simulink model "ControlledVehicleSystem_PID"  (R2019b)
settings: Solver=FixedStepAuto  StartTime=0.0  StopTime=15  FixedStep=0.005  RelTol=1e-3
model workspace (MAT data in the model file):
  I_a = 2.25
  I_f = 2.25
  Kda = 1
  Kdf = 1
  Kpa = 1
  Kpf = 1
  Kpv = 25
  Rfl = 0.1
  Rfr = 0.1
  Rrl = 0.1
  Rrr = 0.1
  Tla = 0.6
  Tlf = 0.6
  coeffDerivative = 1
  m_v = 200
undefined symbols (not defined in the file): DiscIntNeverNeededParam, sigbuilder_block
libraries: simulink x8
settings Model: Creator=arfbj  LastModifiedBy=frqbv

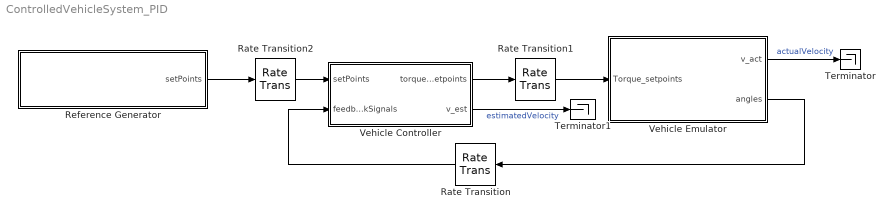
== system ControlledVehicleSystem_PID ==
  Rate Transition : RateTransition
  Rate Transition1 : RateTransition
  Rate Transition2 : RateTransition
  Reference Generator : Subsystem
  Terminator : Terminator
  Terminator1 : Terminator
  Vehicle Controller : Subsystem
  Vehicle Emulator : Subsystem
  wires:
  Vehicle Emulator/2(angles) -> Rate Transition/1
  Reference Generator/1(setPoints) -> Rate Transition2/1
  Vehicle Controller/1(torqueSetpoints) -> Rate Transition1/1
  Vehicle Emulator/1(v_act) -> Terminator/1  "actualVelocity"
  Vehicle Controller/2(v_est) -> Terminator1/1  "estimatedVelocity"
  Rate Transition/1 -> Vehicle Controller/2(feedbackSignals)
  Rate Transition1/1 -> Vehicle Emulator/1(Torque_setpoints)
  Rate Transition2/1 -> Vehicle Controller/1(setPoints)

== system ControlledVehicleSystem_PID/Reference Generator ==
  Bus Creator : BusCreator  Inputs=3
  Signal Builder : Subsystem  Tag=STV Subsys  LoadFcn=sigbuilder_block('load');  StartFcn=sigbuilder_block('start');  StopFcn=sigbuilder_block('stop');  ClipboardFcn=sigbuilder_block('clipboard');  mask(Sigbuilder block){tuvar=[0:10]}
      mask help: Simulink:masks:SigbuilderBlock_MD
      mask init:
      | if ~strcmp(get_param(bdroot(gcbh),'SimulationStatus'),'stopped') tuvar = sigbuilder_block('maskInit'); end
      settings: CopyFcn=sigbuilder_block('copy');  DeleteFcn=sigbuilder_block('delete');  ModelCloseFcn=sigbuilder_block('modelClose');  PreSaveFcn=sigbuilder_block('preSave');  PauseFcn=sigbuilder_block('pause');  ContinueFcn=sigbuilder_block('continue');  NameChangeFcn=sigbuilder_block('namechange');  OpenFcn=sigbuilder_block('open',[1521.6 55.8 550.2 362.4 ]);  CloseFcn=sigbuilder_block('close');
      mask Display: plot(0, 0, 100, 100,[2, 2, 32, 32, 2], [68, 8, 8, 68, 68],[32, 2], [38, 38], [32, 19, 2],[53, 60, 44], [32, 17, 17, 2],[16, 16, 31, 31]);txt = getActiveGroup(gcbh);text(2, 100, txt,'verticalAlignment', 'top');
  setPoints : Outport
  wires:
  Signal Builder/1(v_set) -> Bus Creator/1  "v_set"
  Signal Builder/2(delta_f_set) -> Bus Creator/2  "delta_f_set"
  Signal Builder/3(delta_a_set) -> Bus Creator/3  "delta_a_set"
  Bus Creator/1 -> setPoints/1

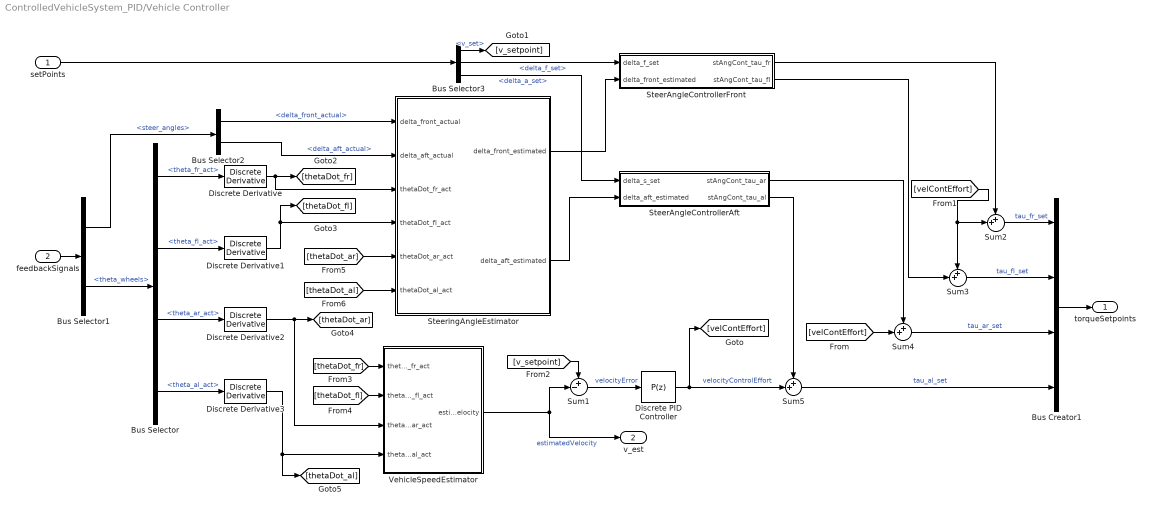
== system ControlledVehicleSystem_PID/Vehicle Controller ==
  setPoints : Inport
  feedbackSignals : Inport  Port=2
  Bus Creator1 : BusCreator  Inputs=4
  Bus Selector : BusSelector  OutputSignals=theta_fr_act,theta_fl_act,theta_ar_act,theta_al_act
  Bus Selector1 : BusSelector  OutputSignals=steer_angles,theta_wheels
  Bus Selector2 : BusSelector  OutputSignals=delta_front_actual,delta_aft_actual
  Bus Selector3 : BusSelector  OutputSignals=v_set,delta_f_set,delta_a_set
  Discrete Derivative{,1..3} (4 alike) : simulink/Discrete/Discrete Derivative  gainval=1.0  ICPrevScaledInput=0.0  OutMin=[]  OutMax=[]  OutDataType=fixdt(1, 16)  OutScaling=2^-10  DoSatur=off
  Discrete PID Controller : simulink/Continuous/PID Controller  Controller=P  Form=Parallel  TimeDomain=Discrete-time  SampleTime=-1  IntegratorMethod=Forward Euler  FilterMethod=Forward Euler  ControllerParametersSource=internal  P=20  I=1  D=5  UseFilter=on  N=100  TunerSelectOption=Transfer Function Based (PID Tuner App)  InitialConditionSource=internal  InitialConditionForIntegrator=0  InitialConditionForFilter=0  DifferentiatorICPrevScaledInput=0  ExternalReset=none  TrackingMode=off  Kt=1  LimitOutput=off  UpperSaturationLimit=inf  LowerSaturationLimit=-inf  LinearizeAsGain=off  AntiWindupMode=none  Kb=1  POutMin=[]  POutMax=[]  IOutMin=[]  IOutMax=[]  DOutMin=[]  DOutMax=[]  NOutMin=[]  NOutMax=[]  SumOutMin=[]  SumOutMax=[]  SaturationOutMin=[]  SaturationOutMax=[]  PParamMin=[]  PParamMax=[]  IParamMin=[]  IParamMax=[]  DParamMin=[]  DParamMax=[]  NParamMin=[]  NParamMax=[]  KbParamMin=[]  KbParamMax=[]  KtParamMin=[]  KtParamMax=[]  KbOutMin=[]  KbOutMax=[]  KtOutMin=[]  KtOutMax=[]  IntegratorOutMin=[]  IntegratorOutMax=[]  FilterOutMin=[]  FilterOutMax=[]  SumI1OutMin=[]  SumI1OutMax=[]  SumI2OutMin=[]  SumI2OutMax=[]  SumI3OutMin=[]  SumI3OutMax=[]  SumI4OutMin=[]  SumI4OutMax=[]  SumDOutMin=[]  SumDOutMax=[]  DifferentiatorOutMin=[]  DifferentiatorOutMax=[]  FilterDiffOutCoefMin=[]  FilterDiffOutCoefMax=[]  ReciprocalOutMin=[]  ReciprocalOutMax=[]  SumDenOutMin=[]  SumDenOutMax=[]  SumNumOutMin=[]  SumNumOutMax=[]  DivideOutMin=[]  DivideOutMax=[]  IntegratorContinuousStateAttributes=''  IntegratorStateMustResolveToSignalObject=off  IntegratorRTWStateStorageClass=Auto  FilterContinuousStateAttributes=''  FilterStateMustResolveToSignalObject=off  FilterRTWStateStorageClass=Auto  ParallelPVariant=InternalParameters  IdealPVariant=Disabled  IVariant=Disabled  DVariant=Disabled  IntegratorVariant=Disabled  SatVariant=Disabled  AWVariant=Disabled  PCopyVariant=Disabled  TRVariant=Disabled  FdbkBlocksVariant=Forward  IdealPFdbkVariant=Disabled  SatFdbkVariant=Disabled  DerivativeFilterVariant=Disabled  NVariant=Disabled  NCopyVariant=Disabled_SignalSpec  FilterICVariant=Disabled  IntegratorICVariant=Disabled  ExternalResetVariant=Disabled  TRSumVariant=Passthrough  SumFdbkVariant=Disabled  SumVariant=Passthrough_P
  SteerAngleControllerAft : Subsystem
  SteerAngleControllerFront : Subsystem
  SteeringAngleEstimator : Subsystem
  Sum1 : Sum  Inputs=+-|
  Sum{2..5} (4 alike) : Sum  Inputs=++|
  VehicleSpeedEstimator : Subsystem
  torqueSetpoints : Outport
  v_est : Outport  Port=2
  wires:
  feedbackSignals/1 -> Bus Selector1/1
  Bus Selector1/2 -> Bus Selector/1  "<theta_wheels>"
  Bus Selector1/1 -> Bus Selector2/1  "<steer_angles>"
  Bus Selector/1 -> Discrete Derivative/1  "<theta_fr_act>"
  Bus Selector/2 -> Discrete Derivative1/1  "<theta_fl_act>"
  Bus Selector/3 -> Discrete Derivative2/1  "<theta_ar_act>"
  Bus Selector/4 -> Discrete Derivative3/1  "<theta_al_act>"
  Discrete Derivative/1 -> [thetaDot_fr], SteeringAngleEstimator/3(thetaDot_fr_act)
  Discrete Derivative2/1 -> VehicleSpeedEstimator/3(thetaDot_ar_act), [thetaDot_ar]
  Discrete Derivative3/1 -> [thetaDot_al], VehicleSpeedEstimator/4(thetaDot_al_act)
  Discrete Derivative1/1 -> [thetaDot_fl], SteeringAngleEstimator/4(thetaDot_fl_act)
  Bus Selector2/1 -> SteeringAngleEstimator/1(delta_front_actual)  "<delta_front_actual>"
  Bus Selector2/2 -> SteeringAngleEstimator/2(delta_aft_actual)  "<delta_aft_actual>"
  SteeringAngleEstimator/1(delta_front_estimated) -> SteerAngleControllerFront/2(delta_front_estimated)
  Bus Creator1/1 -> torqueSetpoints/1
  VehicleSpeedEstimator/1(estimatedVelocity) -> v_est/1, Sum1/2  "estimatedVelocity"
  Sum1/1 -> Discrete PID Controller/1  "velocityError"
  Sum4/1 -> Bus Creator1/3  "tau_ar_set"
  Sum5/1 -> Bus Creator1/4  "tau_al_set"
  Sum3/1 -> Bus Creator1/2  "tau_fl_set"
  Sum2/1 -> Bus Creator1/1  "tau_fr_set"
  setPoints/1 -> Bus Selector3/1
  [v_setpoint] -> Sum1/1
  Bus Selector3/2 -> SteerAngleControllerFront/1(delta_f_set)  "<delta_f_set>"
  SteeringAngleEstimator/2(delta_aft_estimated) -> SteerAngleControllerAft/2(delta_aft_estimated)
  Bus Selector3/3 -> SteerAngleControllerAft/1(delta_s_set)  "<delta_a_set>"
  SteerAngleControllerFront/1(stAngCont_tau_fr) -> Sum2/1
  SteerAngleControllerFront/2(stAngCont_tau_fl) -> Sum3/2
  SteerAngleControllerAft/1(stAngCont_tau_ar) -> Sum4/1
  SteerAngleControllerAft/2(stAngCont_tau_al) -> Sum5/1
  Discrete PID Controller/1 -> [velContEffort], Sum5/2  "velocityControlEffort"
  [velContEffort] -> Sum4/2
  [velContEffort] -> Sum3/1, Sum2/2
  Bus Selector3/1 -> [v_setpoint]  "<v_set>"
  [thetaDot_fr] -> VehicleSpeedEstimator/1(thetaDot_fr_act)
  [thetaDot_fl] -> VehicleSpeedEstimator/2(thetaDot_fl_act)
  [thetaDot_ar] -> SteeringAngleEstimator/5(thetaDot_ar_act)
  [thetaDot_al] -> SteeringAngleEstimator/6(thetaDot_al_act)

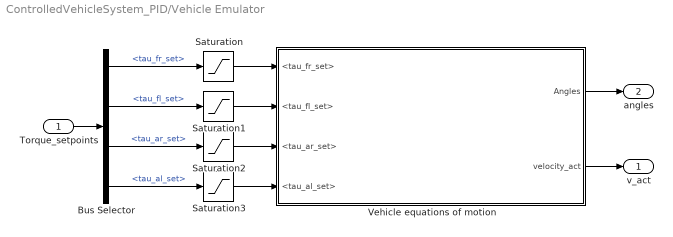
== system ControlledVehicleSystem_PID/Vehicle Emulator ==
  Torque_setpoints : Inport
  Bus Selector : BusSelector  OutputSignals=tau_fr_set,tau_fl_set,tau_ar_set,tau_al_set
  Saturation{,1..3} (4 alike) : Saturate  UpperLimit=5  LowerLimit=-5
  Vehicle equations of motion : Subsystem
  v_act : Outport
  angles : Outport  Port=2
  wires:
  Torque_setpoints/1 -> Bus Selector/1
  Bus Selector/2 -> Saturation1/1  "<tau_fl_set>"
  Bus Selector/1 -> Saturation/1  "<tau_fr_set>"
  Bus Selector/3 -> Saturation2/1  "<tau_ar_set>"
  Bus Selector/4 -> Saturation3/1  "<tau_al_set>"
  Vehicle equations of motion/1(Angles) -> angles/1
  Vehicle equations of motion/2(velocity_act) -> v_act/1
  Saturation/1 -> Vehicle equations of motion/1(<tau_fr_set>)
  Saturation1/1 -> Vehicle equations of motion/2(<tau_fl_set>)
  Saturation2/1 -> Vehicle equations of motion/3(<tau_ar_set>)
  Saturation3/1 -> Vehicle equations of motion/4(<tau_al_set>)

== system ControlledVehicleSystem_PID/Reference Generator/Signal Builder ==
  Demux : Demux  Tag=STV Demux  Outputs=3
  FromWs : FromWorkspace  Tag=STV FromWs  VariableName=tuvar  SampleTime=0
      SigBuilderData=|
      | common.afterFinalStr = 'Extrapolate'
      | common.sampleTime = 0
      | dataSet.timeRange = [0 10]
      | dataSet.name = 'Group 1'
      | sbobj.Groups.Name = 'Group 1'
      | sbobj.Groups.Signals(1).Name = 'v_set'
      | sbobj.Groups.Signals(1).XData = [0 1 3 5 6 8 9 10]
      | sbobj.Groups.Signals(1).YData = [-0.005 -0.00375 1 1 0.5 0.5 0 0]
      | sbobj.Groups.Signals(2).Name = 'delta_f_set'
      | sbobj.Groups.Signals(2).XData = [0 10]
      | sbobj.Groups.Signals(2).YData = [0 0]
      | sbobj.Groups.Signals(3).Name = 'delta_a_set'
      | sbobj.Groups.Signals(3).XData = [0 10]
      | sbobj.Groups.Signals(3).YData = [0 0]
  v_set : Outport  Tag=STV Outport
  delta_f_set : Outport  Tag=STV Outport  Port=2
  delta_a_set : Outport  Tag=STV Outport  Port=3
  wires:
  Demux/1 -> v_set/1
  FromWs/1 -> Demux/1
  Demux/2 -> delta_f_set/1
  Demux/3 -> delta_a_set/1

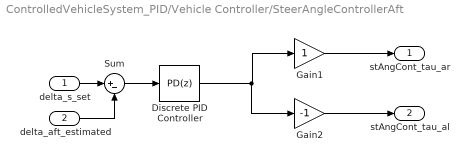
== system ControlledVehicleSystem_PID/Vehicle Controller/SteerAngleControllerAft ==
  delta_s_set : Inport
  delta_aft_estimated : Inport  Port=2
  Discrete PID Controller : simulink/Continuous/PID Controller  Controller=PD  Form=Parallel  TimeDomain=Discrete-time  SampleTime=-1  IntegratorMethod=Forward Euler  FilterMethod=Forward Euler  ControllerParametersSource=internal  P=1  I=1  D=1  UseFilter=on  N=100  TunerSelectOption=Transfer Function Based (PID Tuner App)  InitialConditionSource=internal  InitialConditionForIntegrator=0  InitialConditionForFilter=0  DifferentiatorICPrevScaledInput=0  ExternalReset=none  TrackingMode=off  Kt=1  LimitOutput=off  UpperSaturationLimit=inf  LowerSaturationLimit=-inf  LinearizeAsGain=off  AntiWindupMode=none  Kb=1  POutMin=[]  POutMax=[]  IOutMin=[]  IOutMax=[]  DOutMin=[]  DOutMax=[]  NOutMin=[]  NOutMax=[]  SumOutMin=[]  SumOutMax=[]  SaturationOutMin=[]  SaturationOutMax=[]  PParamMin=[]  PParamMax=[]  IParamMin=[]  IParamMax=[]  DParamMin=[]  DParamMax=[]  NParamMin=[]  NParamMax=[]  KbParamMin=[]  KbParamMax=[]  KtParamMin=[]  KtParamMax=[]  KbOutMin=[]  KbOutMax=[]  KtOutMin=[]  KtOutMax=[]  IntegratorOutMin=[]  IntegratorOutMax=[]  FilterOutMin=[]  FilterOutMax=[]  SumI1OutMin=[]  SumI1OutMax=[]  SumI2OutMin=[]  SumI2OutMax=[]  SumI3OutMin=[]  SumI3OutMax=[]  SumI4OutMin=[]  SumI4OutMax=[]  SumDOutMin=[]  SumDOutMax=[]  DifferentiatorOutMin=[]  DifferentiatorOutMax=[]  FilterDiffOutCoefMin=[]  FilterDiffOutCoefMax=[]  ReciprocalOutMin=[]  ReciprocalOutMax=[]  SumDenOutMin=[]  SumDenOutMax=[]  SumNumOutMin=[]  SumNumOutMax=[]  DivideOutMin=[]  DivideOutMax=[]  IntegratorContinuousStateAttributes=''  IntegratorStateMustResolveToSignalObject=off  IntegratorRTWStateStorageClass=Auto  FilterContinuousStateAttributes=''  FilterStateMustResolveToSignalObject=off  FilterRTWStateStorageClass=Auto  ParallelPVariant=InternalParameters  IdealPVariant=Disabled  IVariant=Disabled  DVariant=InternalParameters  IntegratorVariant=Disabled  SatVariant=Disabled  AWVariant=Disabled  PCopyVariant=Disabled  TRVariant=Disabled  FdbkBlocksVariant=Forward  IdealPFdbkVariant=Disabled  SatFdbkVariant=Disabled  DerivativeFilterVariant=ForwardEulerFilter  NVariant=InternalParameters  NCopyVariant=Disabled  FilterICVariant=InternalICsFilter  IntegratorICVariant=Disabled  ExternalResetVariant=Disabled  TRSumVariant=Passthrough  SumFdbkVariant=Disabled  SumVariant=Sum_PD
  Gain1 : Gain
  Gain2 : Gain  Gain=-1
  Sum : Sum  Inputs=|+-
  stAngCont_tau_ar : Outport
  stAngCont_tau_al : Outport  Port=2
  wires:
  Gain1/1 -> stAngCont_tau_ar/1
  Gain2/1 -> stAngCont_tau_al/1
  delta_s_set/1 -> Sum/1
  Sum/1 -> Discrete PID Controller/1
  delta_aft_estimated/1 -> Sum/2
  Discrete PID Controller/1 -> Gain2/1, Gain1/1

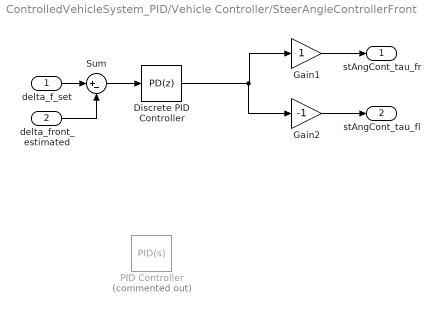
== system ControlledVehicleSystem_PID/Vehicle Controller/SteerAngleControllerFront ==
  delta_f_set : Inport
  delta_front_estimated : Inport  Port=2
  Discrete PID Controller : simulink/Continuous/PID Controller  Controller=PD  Form=Parallel  TimeDomain=Discrete-time  SampleTime=-1  IntegratorMethod=Forward Euler  FilterMethod=Forward Euler  ControllerParametersSource=internal  P=1  I=0  D=1  UseFilter=on  N=100  TunerSelectOption=Transfer Function Based (PID Tuner App)  InitialConditionSource=internal  InitialConditionForIntegrator=0  InitialConditionForFilter=0  DifferentiatorICPrevScaledInput=0  ExternalReset=none  TrackingMode=off  Kt=1  LimitOutput=off  UpperSaturationLimit=inf  LowerSaturationLimit=-inf  LinearizeAsGain=off  AntiWindupMode=none  Kb=1  POutMin=[]  POutMax=[]  IOutMin=[]  IOutMax=[]  DOutMin=[]  DOutMax=[]  NOutMin=[]  NOutMax=[]  SumOutMin=[]  SumOutMax=[]  SaturationOutMin=[]  SaturationOutMax=[]  PParamMin=[]  PParamMax=[]  IParamMin=[]  IParamMax=[]  DParamMin=[]  DParamMax=[]  NParamMin=[]  NParamMax=[]  KbParamMin=[]  KbParamMax=[]  KtParamMin=[]  KtParamMax=[]  KbOutMin=[]  KbOutMax=[]  KtOutMin=[]  KtOutMax=[]  IntegratorOutMin=[]  IntegratorOutMax=[]  FilterOutMin=[]  FilterOutMax=[]  SumI1OutMin=[]  SumI1OutMax=[]  SumI2OutMin=[]  SumI2OutMax=[]  SumI3OutMin=[]  SumI3OutMax=[]  SumI4OutMin=[]  SumI4OutMax=[]  SumDOutMin=[]  SumDOutMax=[]  DifferentiatorOutMin=[]  DifferentiatorOutMax=[]  FilterDiffOutCoefMin=[]  FilterDiffOutCoefMax=[]  ReciprocalOutMin=[]  ReciprocalOutMax=[]  SumDenOutMin=[]  SumDenOutMax=[]  SumNumOutMin=[]  SumNumOutMax=[]  DivideOutMin=[]  DivideOutMax=[]  IntegratorContinuousStateAttributes=''  IntegratorStateMustResolveToSignalObject=off  IntegratorRTWStateStorageClass=Auto  FilterContinuousStateAttributes=''  FilterStateMustResolveToSignalObject=off  FilterRTWStateStorageClass=Auto  ParallelPVariant=InternalParameters  IdealPVariant=Disabled  IVariant=Disabled  DVariant=InternalParameters  IntegratorVariant=Disabled  SatVariant=Disabled  AWVariant=Disabled  PCopyVariant=Disabled  TRVariant=Disabled  FdbkBlocksVariant=Forward  IdealPFdbkVariant=Disabled  SatFdbkVariant=Disabled  DerivativeFilterVariant=ForwardEulerFilter  NVariant=InternalParameters  NCopyVariant=Disabled  FilterICVariant=InternalICsFilter  IntegratorICVariant=Disabled  ExternalResetVariant=Disabled  TRSumVariant=Passthrough  SumFdbkVariant=Disabled  SumVariant=Sum_PD
  Gain1 : Gain
  Gain2 : Gain  Gain=-1
  PID Controller : simulink/Continuous/PID Controller  Commented=on  Controller=PID  Form=Parallel  TimeDomain=Continuous-time  SampleTime=-1  IntegratorMethod=Forward Euler  FilterMethod=Forward Euler  ControllerParametersSource=internal  P=Kpf  I=1  D=Kdf  UseFilter=on  N=100  TunerSelectOption=Transfer Function Based (PID Tuner App)  InitialConditionSource=internal  InitialConditionForIntegrator=0  InitialConditionForFilter=0  DifferentiatorICPrevScaledInput=0  ExternalReset=none  TrackingMode=off  Kt=1  LimitOutput=off  UpperSaturationLimit=inf  LowerSaturationLimit=-inf  LinearizeAsGain=on  AntiWindupMode=none  Kb=1  POutMin=[]  POutMax=[]  IOutMin=[]  IOutMax=[]  DOutMin=[]  DOutMax=[]  NOutMin=[]  NOutMax=[]  SumOutMin=[]  SumOutMax=[]  SaturationOutMin=[]  SaturationOutMax=[]  PParamMin=[]  PParamMax=[]  IParamMin=[]  IParamMax=[]  DParamMin=[]  DParamMax=[]  NParamMin=[]  NParamMax=[]  KbParamMin=[]  KbParamMax=[]  KtParamMin=[]  KtParamMax=[]  KbOutMin=[]  KbOutMax=[]  KtOutMin=[]  KtOutMax=[]  IntegratorOutMin=[]  IntegratorOutMax=[]  FilterOutMin=[]  FilterOutMax=[]  SumI1OutMin=[]  SumI1OutMax=[]  SumI2OutMin=[]  SumI2OutMax=[]  SumI3OutMin=[]  SumI3OutMax=[]  SumI4OutMin=[]  SumI4OutMax=[]  SumDOutMin=[]  SumDOutMax=[]  DifferentiatorOutMin=[]  DifferentiatorOutMax=[]  FilterDiffOutCoefMin=[]  FilterDiffOutCoefMax=[]  ReciprocalOutMin=[]  ReciprocalOutMax=[]  SumDenOutMin=[]  SumDenOutMax=[]  SumNumOutMin=[]  SumNumOutMax=[]  DivideOutMin=[]  DivideOutMax=[]  IntegratorContinuousStateAttributes=''  IntegratorStateMustResolveToSignalObject=off  IntegratorRTWStateStorageClass=Auto  FilterContinuousStateAttributes=''  FilterStateMustResolveToSignalObject=off  FilterRTWStateStorageClass=Auto  ParallelPVariant=InternalParameters  IdealPVariant=Disabled  IVariant=InternalParameters  DVariant=InternalParameters  IntegratorVariant=Continuous  SatVariant=Disabled  AWVariant=Passthrough  PCopyVariant=Disabled  TRVariant=Disabled  FdbkBlocksVariant=Forward  IdealPFdbkVariant=Disabled  SatFdbkVariant=Disabled  DerivativeFilterVariant=ContFilter  NVariant=InternalParameters  NCopyVariant=Disabled  FilterICVariant=InternalICsFilter  IntegratorICVariant=InternalICs  ExternalResetVariant=Disabled  TRSumVariant=Passthrough  SumFdbkVariant=Disabled  SumVariant=Sum_PID
  Sum : Sum  Inputs=|+-
  stAngCont_tau_fr : Outport
  stAngCont_tau_fl : Outport  Port=2
  wires:
  Discrete PID Controller/1 -> Gain2/1, Gain1/1
  Gain1/1 -> stAngCont_tau_fr/1
  Gain2/1 -> stAngCont_tau_fl/1
  delta_f_set/1 -> Sum/1
  Sum/1 -> Discrete PID Controller/1
  delta_front_estimated/1 -> Sum/2

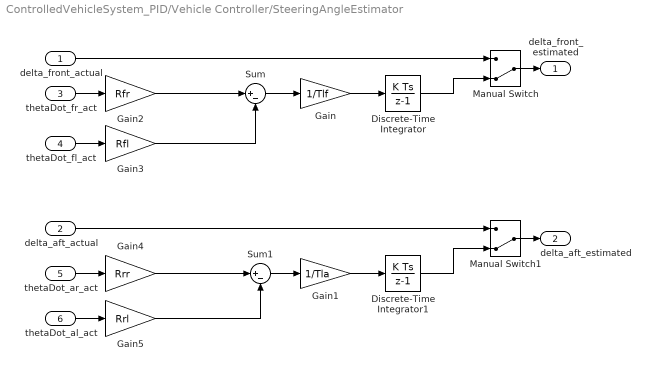
== system ControlledVehicleSystem_PID/Vehicle Controller/SteeringAngleEstimator ==
  delta_front_actual : Inport
  delta_aft_actual : Inport  Port=2
  thetaDot_fr_act : Inport  Port=3
  thetaDot_fl_act : Inport  Port=4
  thetaDot_ar_act : Inport  Port=5
  thetaDot_al_act : Inport  Port=6
  Discrete-Time Integrator : DiscreteIntegrator  SampleTime=-1  ICPrevOutput=DiscIntNeverNeededParam  ICPrevScaledInput=DiscIntNeverNeededParam
  Discrete-Time Integrator1 : DiscreteIntegrator  SampleTime=-1  ICPrevOutput=DiscIntNeverNeededParam  ICPrevScaledInput=DiscIntNeverNeededParam
  Gain : Gain  Gain=1/Tlf
  Gain1 : Gain  Gain=1/Tla
  Gain2 : Gain  Gain=Rfr
  Gain3 : Gain  Gain=Rfl
  Gain4 : Gain  Gain=Rrr
  Gain5 : Gain  Gain=Rrl
  Manual Switch : ManualSwitch  CurrentSetting=0
  Manual Switch1 : ManualSwitch  CurrentSetting=0
  Sum : Sum  Inputs=|+-
  Sum1 : Sum  Inputs=|+-
  delta_front_estimated : Outport
  delta_aft_estimated : Outport  Port=2
  wires:
  Gain/1 -> Discrete-Time Integrator/1
  Discrete-Time Integrator/1 -> Manual Switch/2
  Gain1/1 -> Discrete-Time Integrator1/1
  Manual Switch/1 -> delta_front_estimated/1
  Discrete-Time Integrator1/1 -> Manual Switch1/2
  thetaDot_fr_act/1 -> Gain2/1
  delta_front_actual/1 -> Manual Switch/1
  thetaDot_al_act/1 -> Gain5/1
  Sum1/1 -> Gain1/1
  Sum/1 -> Gain/1
  thetaDot_ar_act/1 -> Gain4/1
  thetaDot_fl_act/1 -> Gain3/1
  delta_aft_actual/1 -> Manual Switch1/1
  Manual Switch1/1 -> delta_aft_estimated/1
  Gain2/1 -> Sum/1
  Gain3/1 -> Sum/2
  Gain4/1 -> Sum1/1
  Gain5/1 -> Sum1/2

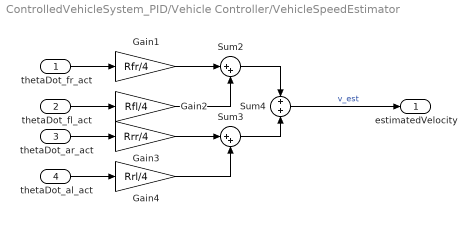
== system ControlledVehicleSystem_PID/Vehicle Controller/VehicleSpeedEstimator ==
  thetaDot_fr_act : Inport
  thetaDot_fl_act : Inport  Port=2
  thetaDot_ar_act : Inport  Port=3
  thetaDot_al_act : Inport  Port=4
  Gain1 : Gain  Gain=Rfr/4
  Gain2 : Gain  Gain=Rfl/4
  Gain3 : Gain  Gain=Rrr/4
  Gain4 : Gain  Gain=Rrl/4
  Sum2 : Sum  Inputs=|++
  Sum3 : Sum  Inputs=|++
  Sum4 : Sum  Inputs=+|+
  estimatedVelocity : Outport
  wires:
  thetaDot_al_act/1 -> Gain4/1
  Sum3/1 -> Sum4/2
  thetaDot_ar_act/1 -> Gain3/1
  Sum2/1 -> Sum4/1
  thetaDot_fl_act/1 -> Gain2/1
  thetaDot_fr_act/1 -> Gain1/1
  Sum4/1 -> estimatedVelocity/1  "v_est"
  Gain1/1 -> Sum2/1
  Gain2/1 -> Sum2/2
  Gain3/1 -> Sum3/1
  Gain4/1 -> Sum3/2

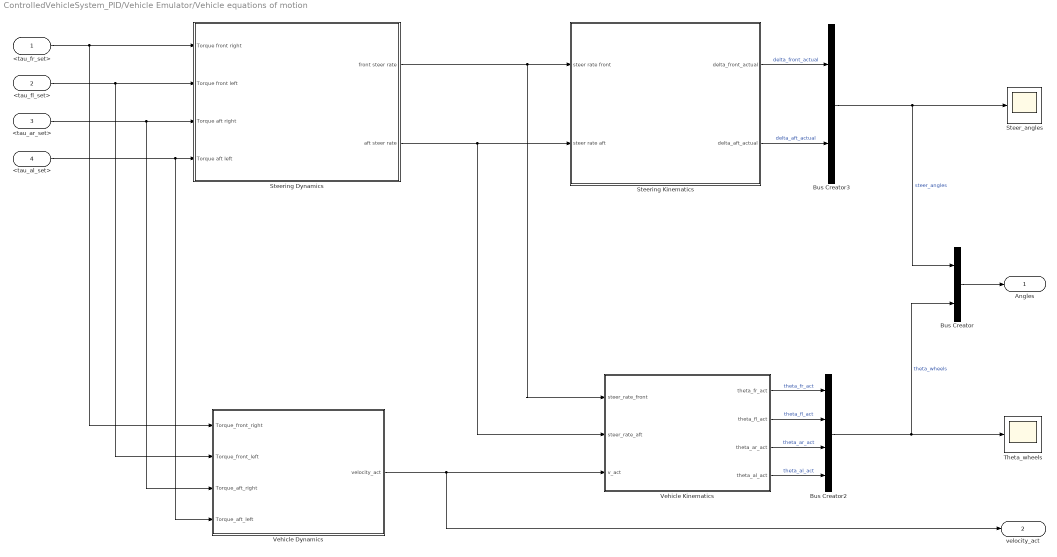
== system ControlledVehicleSystem_PID/Vehicle Emulator/Vehicle equations of motion ==
  <tau_fr_set> : Inport
  <tau_fl_set> : Inport  Port=2
  <tau_ar_set> : Inport  Port=3
  <tau_al_set> : Inport  Port=4
  Bus Creator : BusCreator  Inputs=2
  Bus Creator2 : BusCreator  Inputs=4
  Bus Creator3 : BusCreator  Inputs=2
  Steer_angles : Scope
  Steering Dynamics : Subsystem
  Steering Kinematics : Subsystem
  Theta_wheels : Scope
  Vehicle Dynamics : Subsystem
  Vehicle Kinematics : Subsystem
  Angles : Outport
  velocity_act : Outport  Port=2
  wires:
  Steering Kinematics/2(delta_aft_actual) -> Bus Creator3/2  "delta_aft_actual"
  Bus Creator3/1 -> Bus Creator/1, Steer_angles/1  "steer_angles"
  Steering Kinematics/1(delta_front_actual) -> Bus Creator3/1  "delta_front_actual"
  <tau_al_set>/1 -> Vehicle Dynamics/4(Torque_aft_left), Steering Dynamics/4(Torque aft left)
  <tau_ar_set>/1 -> Vehicle Dynamics/3(Torque_aft_right), Steering Dynamics/3(Torque aft right)
  <tau_fr_set>/1 -> Vehicle Dynamics/1(Torque_front_right), Steering Dynamics/1(Torque front right)
  <tau_fl_set>/1 -> Vehicle Dynamics/2(Torque_front_left), Steering Dynamics/2(Torque front left)
  Vehicle Kinematics/1(theta_fr_act) -> Bus Creator2/1  "theta_fr_act"
  Vehicle Kinematics/2(theta_fl_act) -> Bus Creator2/2  "theta_fl_act"
  Vehicle Kinematics/3(theta_ar_act) -> Bus Creator2/3  "theta_ar_act"
  Vehicle Kinematics/4(theta_al_act) -> Bus Creator2/4  "theta_al_act"
  Bus Creator2/1 -> Bus Creator/2, Theta_wheels/1  "theta_wheels"
  Bus Creator/1 -> Angles/1
  Vehicle Dynamics/1(velocity_act) -> velocity_act/1, Vehicle Kinematics/3(v_act)
  Steering Dynamics/1(front steer rate) -> Vehicle Kinematics/1(steer_rate_front), Steering Kinematics/1(steer rate front)
  Steering Dynamics/2(aft steer rate) -> Vehicle Kinematics/2(steer_rate_aft), Steering Kinematics/2(steer rate aft)

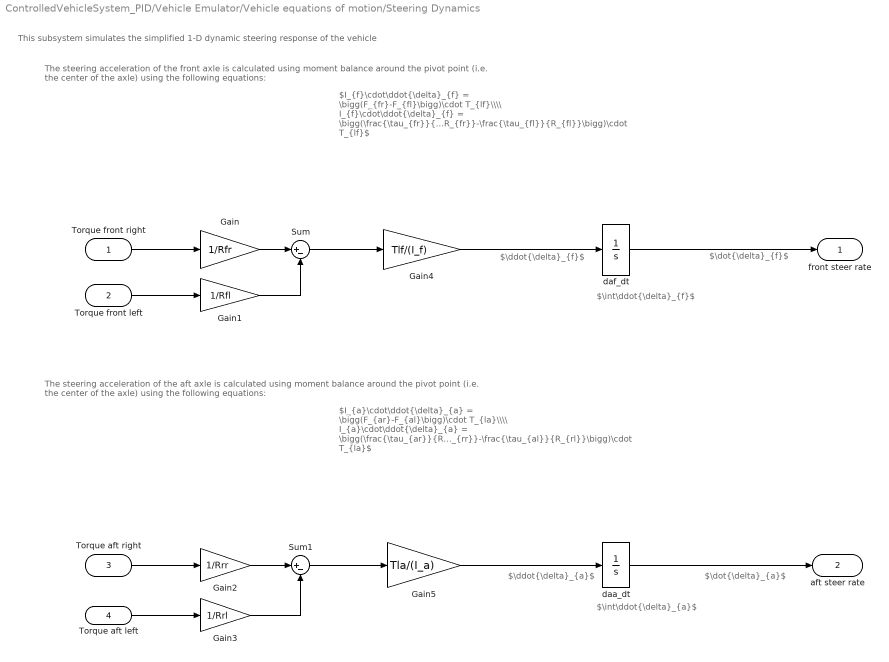
== system ControlledVehicleSystem_PID/Vehicle Emulator/Vehicle equations of motion/Steering Dynamics ==
  note: This subsystem simulates the simplified 1-D dynamic steering response of the vehicle
  note: $\int\ddot{\delta}_{f}$
  note: $\ddot{\delta}_{f}$
  note: $I_{f}\cdot\ddot{\delta}_{f} = \bigg(F_{fr}-F_{fl}\bigg)\cdot T_{lf}\\\\ I_{f}\cdot\ddot{\delta}_{f} = \bigg(\frac{\tau_{fr}}{R_{fr}}-\frac{\tau_{fl}}{R_{fl}}\bigg)\cdot T_{lf}$
  note: The steering acceleration of the front axle is calculated using moment balance around the pivot point (i.e. the center of the axle) using the following equations:
  note: $I_{a}\cdot\ddot{\delta}_{a} = \bigg(F_{ar}-F_{al}\bigg)\cdot T_{la}\\\\ I_{a}\cdot\ddot{\delta}_{a} = \bigg(\frac{\tau_{ar}}{R_{rr}}-\frac{\tau_{al}}{R_{rl}}\bigg)\cdot T_{la}$
  note: The steering acceleration of the aft axle is calculated using moment balance around the pivot point (i.e. the center of the axle) using the following equations:
  note: $\dot{\delta}_{f}$
  note: $\ddot{\delta}_{a}$
  note: $\dot{\delta}_{a}$
  note: $\int\ddot{\delta}_{a}$
  Torque front right : Inport
  Torque front left : Inport  Port=2
  Torque aft right : Inport  Port=3
  Torque aft left : Inport  Port=4
  Gain : Gain  Gain=1/Rfr
  Gain1 : Gain  Gain=1/Rfl
  Gain2 : Gain  Gain=1/Rrr
  Gain3 : Gain  Gain=1/Rrl
  Gain4 : Gain  Gain=Tlf/(I_f)
  Gain5 : Gain  Gain=Tla/(I_a)
  Sum : Sum  Inputs=|+-
  Sum1 : Sum  Inputs=|+-
  daa_dt : Integrator
  daf_dt : Integrator
  front steer rate : Outport
  aft steer rate : Outport  Port=2
  wires:
  daa_dt/1 -> aft steer rate/1
  Torque aft left/1 -> Gain3/1
  Torque aft right/1 -> Gain2/1
  Sum/1 -> Gain4/1
  Gain5/1 -> daa_dt/1
  Torque front left/1 -> Gain1/1
  daf_dt/1 -> front steer rate/1
  Gain4/1 -> daf_dt/1
  Sum1/1 -> Gain5/1
  Torque front right/1 -> Gain/1
  Gain/1 -> Sum/1
  Gain1/1 -> Sum/2
  Gain2/1 -> Sum1/1
  Gain3/1 -> Sum1/2

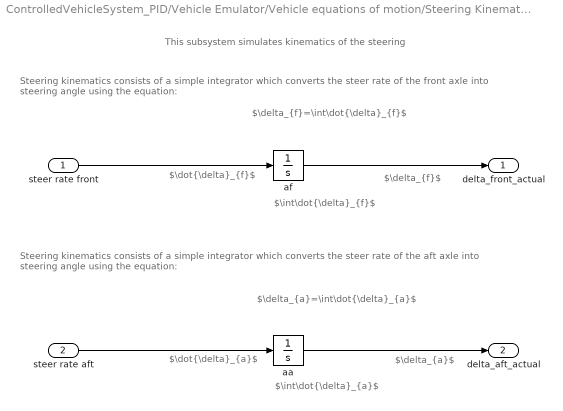
== system ControlledVehicleSystem_PID/Vehicle Emulator/Vehicle equations of motion/Steering Kinematics ==
  note: $\delta_{f}=\int\dot{\delta}_{f}$
  note: Steering kinematics consists of a simple integrator which converts the steer rate of the front axle into steering
      | angle using the equation:
  note: $\int\dot{\delta}_{f}$
  note: $\delta_{f}$
  note: $\dot{\delta}_{f}$
  note: This subsystem simulates kinematics of the steering
  note: $\dot{\delta}_{a}$
  note: $\int\dot{\delta}_{a}$
  note: $\delta_{a}$
  note: Steering kinematics consists of a simple integrator which converts the steer rate of the aft axle into steering
      | angle using the equation:
  note: $\delta_{a}=\int\dot{\delta}_{a}$
  steer rate front : Inport
  steer rate aft : Inport  Port=2
  aa : Integrator  InitialCondition=-0.2
  af : Integrator  InitialCondition=0.1
  delta_front_actual : Outport
  delta_aft_actual : Outport  Port=2
  wires:
  af/1 -> delta_front_actual/1
  steer rate front/1 -> af/1
  aa/1 -> delta_aft_actual/1
  steer rate aft/1 -> aa/1

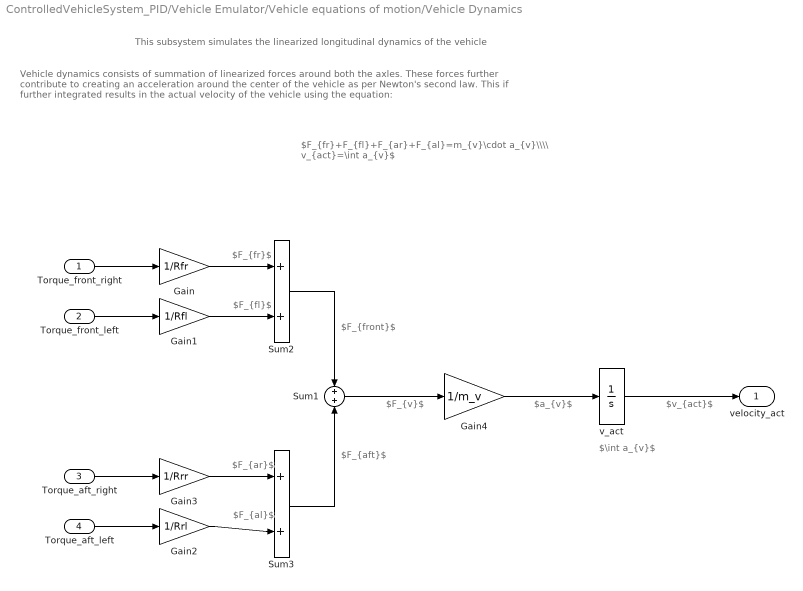
== system ControlledVehicleSystem_PID/Vehicle Emulator/Vehicle equations of motion/Vehicle Dynamics ==
  note: $F_{front}$
  note: $F_{fr}+F_{fl}+F_{ar}+F_{al}=m_{v}\cdot a_{v}\\\\ v_{act}=\int a_{v}$
  note: Vehicle dynamics consists of summation of linearized forces around both the axles. These forces further contribute to creating an
      | acceleration around the center of the vehicle as per Newton's second law. This if further integrated results in the actual velocity of the
      | vehicle using the equation:
  note: This subsystem simulates the linearized longitudinal dynamics of the vehicle
  note: $F_{aft}$
  note: $F_{v}$
  note: $a_{v}$
  note: $\int a_{v}$
  note: $v_{act}$
  note: $F_{fr}$
  note: $F_{fl}$
  note: $F_{ar}$
  note: $F_{al}$
  Torque_front_right : Inport
  Torque_front_left : Inport  Port=2
  Torque_aft_right : Inport  Port=3
  Torque_aft_left : Inport  Port=4
  Gain : Gain  Gain=1/Rfr
  Gain1 : Gain  Gain=1/Rfl
  Gain2 : Gain  Gain=1/Rrl
  Gain3 : Gain  Gain=1/Rrr
  Gain4 : Gain  Gain=1/m_v
  Sum1 : Sum
  Sum2 : Sum
  Sum3 : Sum
  v_act : Integrator
  velocity_act : Outport
  wires:
  Torque_front_left/1 -> Gain1/1
  Torque_front_right/1 -> Gain/1
  Sum1/1 -> Gain4/1
  v_act/1 -> velocity_act/1
  Sum3/1 -> Sum1/2
  Torque_aft_right/1 -> Gain3/1
  Gain4/1 -> v_act/1
  Sum2/1 -> Sum1/1
  Torque_aft_left/1 -> Gain2/1
  Gain/1 -> Sum2/1
  Gain1/1 -> Sum2/2
  Gain2/1 -> Sum3/2
  Gain3/1 -> Sum3/1

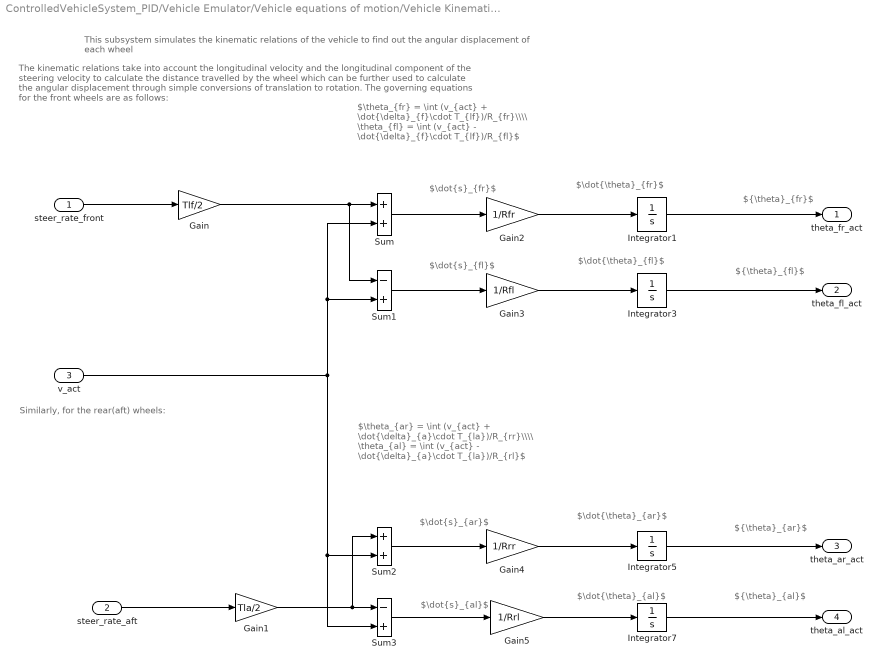
== system ControlledVehicleSystem_PID/Vehicle Emulator/Vehicle equations of motion/Vehicle Kinematics ==
  note: $\dot{s}_{fr}$
  note: Similarly, for the rear(aft) wheels:
  note: $\theta_{fr} = \int (v_{act} + \dot{\delta}_{f}\cdot T_{lf})/R_{fr}\\\\ \theta_{fl} = \int (v_{act} - \dot{\delta}_{f}\cdot T_{lf})/R_{fl}$
  note: The kinematic relations take into account the longitudinal velocity and the longitudinal component of the steering velocity to calculate the distance travelled by
      | the wheel which can be further used to calculate the angular displacement through simple conversions of translation to rotation. The governing equations for
      | the front wheels are as follows:
  note: This subsystem simulates the kinematic relations of the vehicle to find out the angular displacement of each wheel
  note: $\theta_{ar} = \int (v_{act} + \dot{\delta}_{a}\cdot T_{la})/R_{rr}\\\\ \theta_{al} = \int (v_{act} - \dot{\delta}_{a}\cdot T_{la})/R_{rl}$
  note: $\dot{s}_{fl}$
  note: $\dot{s}_{ar}$
  note: $\dot{s}_{al}$
  note: $\dot{\theta}_{fr}$
  note: $\dot{\theta}_{fl}$
  note: $\dot{\theta}_{ar}$
  note: $\dot{\theta}_{al}$
  note: ${\theta}_{fr}$
  note: ${\theta}_{fl}$
  note: ${\theta}_{ar}$
  note: ${\theta}_{al}$
  steer_rate_front : Inport
  steer_rate_aft : Inport  Port=2
  v_act : Inport  Port=3
  Gain : Gain  Gain=Tlf/2
  Gain1 : Gain  Gain=Tla/2
  Gain2 : Gain  Gain=1/Rfr
  Gain3 : Gain  Gain=1/Rfl
  Gain4 : Gain  Gain=1/Rrr
  Gain5 : Gain  Gain=1/Rrl
  Integrator{1,3,5,7} (4 alike) : Integrator
  Sum : Sum
  Sum1 : Sum  Inputs=-+
  Sum2 : Sum
  Sum3 : Sum  Inputs=-+
  theta_fr_act : Outport
  theta_fl_act : Outport  Port=2
  theta_ar_act : Outport  Port=3
  theta_al_act : Outport  Port=4
  wires:
  Integrator1/1 -> theta_fr_act/1
  Integrator3/1 -> theta_fl_act/1
  Integrator5/1 -> theta_ar_act/1
  Integrator7/1 -> theta_al_act/1
  steer_rate_front/1 -> Gain/1
  steer_rate_aft/1 -> Gain1/1
  Gain/1 -> Sum1/1, Sum/1
  Sum/1 -> Gain2/1
  Sum1/1 -> Gain3/1
  Sum3/1 -> Gain5/1
  Sum2/1 -> Gain4/1
  Gain1/1 -> Sum3/1, Sum2/1
  v_act/1 -> Sum/2, Sum1/2, Sum2/2, Sum3/2
  Gain2/1 -> Integrator1/1
  Gain3/1 -> Integrator3/1
  Gain4/1 -> Integrator5/1
  Gain5/1 -> Integrator7/1
